simulink model "motor_new"  (R2018b)
settings: Solver=FixedStepAuto  StartTime=0.0  StopTime=100  FixedStep=0.001  RelTol=1e-3
values from neighbouring files (symbols this model uses):
  wt = 20    [Para_new.m]
libraries: simulink x2
settings Model: Creator=chengqian  LastModifiedBy=chengqian
settings SolverCC: AlgebraicLoopSolver=LineSearch

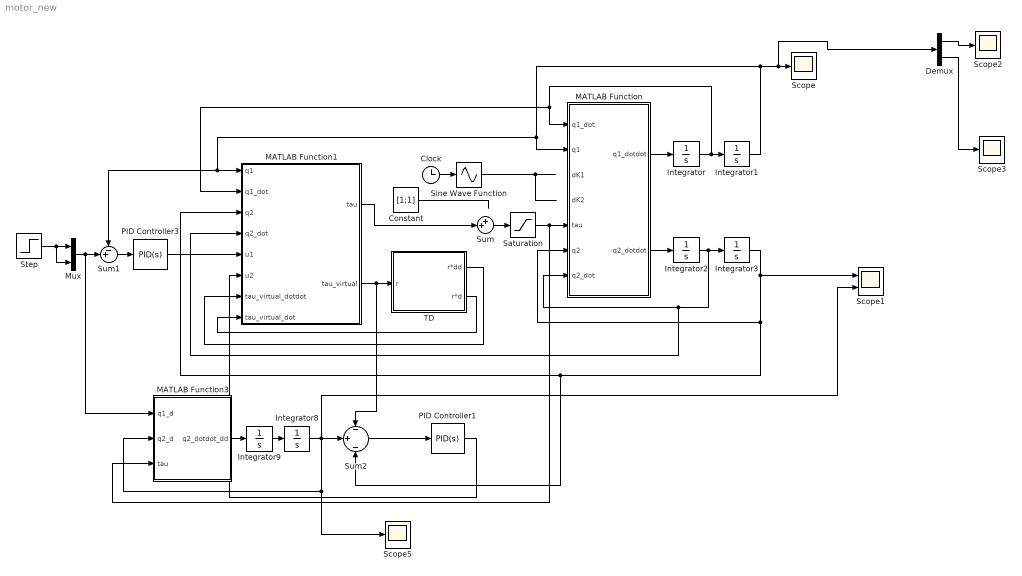
== system motor_new ==
  Clock : Clock
  Constant : Constant  Value=[1;1]
  Demux : Demux  Outputs=2
  Integrator{,1..3,8..9} (6 alike) : Integrator
  MATLAB Function : MATLAB Function  TreatAsAtomicUnit=on
  MATLAB Function1 : MATLAB Function  TreatAsAtomicUnit=on
  MATLAB Function3 : MATLAB Function  TreatAsAtomicUnit=on
  Mux : Mux  Inputs=2
  PID Controller1 : simulink/Continuous/PID Controller  Controller=PID  Form=Parallel  TimeDomain=Continuous-time  SampleTime=-1  IntegratorMethod=Forward Euler  FilterMethod=Forward Euler  ControllerParametersSource=internal  P=[0;0]  I=[0;0]  D=[0;0]  UseFilter=on  N=1000  TunerSelectOption=Transfer Function Based (PID Tuner App)  InitialConditionSource=internal  InitialConditionForIntegrator=0  InitialConditionForFilter=0  DifferentiatorICPrevScaledInput=0  ExternalReset=none  TrackingMode=off  Kt=1  LimitOutput=off  UpperSaturationLimit=inf  LowerSaturationLimit=-inf  LinearizeAsGain=on  AntiWindupMode=none  Kb=1  POutMin=[]  POutMax=[]  IOutMin=[]  IOutMax=[]  DOutMin=[]  DOutMax=[]  NOutMin=[]  NOutMax=[]  SumOutMin=[]  SumOutMax=[]  SaturationOutMin=[]  SaturationOutMax=[]  PParamMin=[]  PParamMax=[]  IParamMin=[]  IParamMax=[]  DParamMin=[]  DParamMax=[]  NParamMin=[]  NParamMax=[]  KbParamMin=[]  KbParamMax=[]  KtParamMin=[]  KtParamMax=[]  KbOutMin=[]  KbOutMax=[]  KtOutMin=[]  KtOutMax=[]  IntegratorOutMin=[]  IntegratorOutMax=[]  FilterOutMin=[]  FilterOutMax=[]  SumI1OutMin=[]  SumI1OutMax=[]  SumI2OutMin=[]  SumI2OutMax=[]  SumI3OutMin=[]  SumI3OutMax=[]  SumI4OutMin=[]  SumI4OutMax=[]  SumDOutMin=[]  SumDOutMax=[]  DifferentiatorOutMin=[]  DifferentiatorOutMax=[]  FilterDiffOutCoefMin=[]  FilterDiffOutCoefMax=[]  ReciprocalOutMin=[]  ReciprocalOutMax=[]  SumDenOutMin=[]  SumDenOutMax=[]  SumNumOutMin=[]  SumNumOutMax=[]  DivideOutMin=[]  DivideOutMax=[]  IntegratorContinuousStateAttributes=''  IntegratorStateMustResolveToSignalObject=off  IntegratorRTWStateStorageClass=Auto  FilterContinuousStateAttributes=''  FilterStateMustResolveToSignalObject=off  FilterRTWStateStorageClass=Auto  ParallelPVariant=InternalParameters  IdealPVariant=Disabled  IVariant=InternalParameters  DVariant=InternalParameters  IntegratorVariant=Continuous  SatVariant=Disabled  AWVariant=Passthrough  PCopyVariant=Disabled  TRVariant=Disabled  FdbkBlocksVariant=Forward  IdealPFdbkVariant=Disabled  SatFdbkVariant=Disabled  DerivativeFilterVariant=ContFilter  NVariant=InternalParameters  NCopyVariant=Disabled  FilterICVariant=InternalICsFilter  IntegratorICVariant=InternalICs  ExternalResetVariant=Disabled  TRSumVariant=Passthrough  SumFdbkVariant=Disabled  SumVariant=Sum_PID
  PID Controller3 : simulink/Continuous/PID Controller  Controller=PID  Form=Parallel  TimeDomain=Continuous-time  SampleTime=-1  IntegratorMethod=Forward Euler  FilterMethod=Forward Euler  ControllerParametersSource=internal  P=[2;2]  I=[0;0]  D=[0.1;0.05]  UseFilter=on  N=1000  TunerSelectOption=Transfer Function Based (PID Tuner App)  InitialConditionSource=internal  InitialConditionForIntegrator=0  InitialConditionForFilter=0  DifferentiatorICPrevScaledInput=0  ExternalReset=none  TrackingMode=off  Kt=1  LimitOutput=off  UpperSaturationLimit=inf  LowerSaturationLimit=-inf  LinearizeAsGain=on  AntiWindupMode=none  Kb=1  POutMin=[]  POutMax=[]  IOutMin=[]  IOutMax=[]  DOutMin=[]  DOutMax=[]  NOutMin=[]  NOutMax=[]  SumOutMin=[]  SumOutMax=[]  SaturationOutMin=[]  SaturationOutMax=[]  PParamMin=[]  PParamMax=[]  IParamMin=[]  IParamMax=[]  DParamMin=[]  DParamMax=[]  NParamMin=[]  NParamMax=[]  KbParamMin=[]  KbParamMax=[]  KtParamMin=[]  KtParamMax=[]  KbOutMin=[]  KbOutMax=[]  KtOutMin=[]  KtOutMax=[]  IntegratorOutMin=[]  IntegratorOutMax=[]  FilterOutMin=[]  FilterOutMax=[]  SumI1OutMin=[]  SumI1OutMax=[]  SumI2OutMin=[]  SumI2OutMax=[]  SumI3OutMin=[]  SumI3OutMax=[]  SumI4OutMin=[]  SumI4OutMax=[]  SumDOutMin=[]  SumDOutMax=[]  DifferentiatorOutMin=[]  DifferentiatorOutMax=[]  FilterDiffOutCoefMin=[]  FilterDiffOutCoefMax=[]  ReciprocalOutMin=[]  ReciprocalOutMax=[]  SumDenOutMin=[]  SumDenOutMax=[]  SumNumOutMin=[]  SumNumOutMax=[]  DivideOutMin=[]  DivideOutMax=[]  IntegratorContinuousStateAttributes=''  IntegratorStateMustResolveToSignalObject=off  IntegratorRTWStateStorageClass=Auto  FilterContinuousStateAttributes=''  FilterStateMustResolveToSignalObject=off  FilterRTWStateStorageClass=Auto  ParallelPVariant=InternalParameters  IdealPVariant=Disabled  IVariant=InternalParameters  DVariant=InternalParameters  IntegratorVariant=Continuous  SatVariant=Disabled  AWVariant=Passthrough  PCopyVariant=Disabled  TRVariant=Disabled  FdbkBlocksVariant=Forward  IdealPFdbkVariant=Disabled  SatFdbkVariant=Disabled  DerivativeFilterVariant=ContFilter  NVariant=InternalParameters  NCopyVariant=Disabled  FilterICVariant=InternalICsFilter  IntegratorICVariant=InternalICs  ExternalResetVariant=Disabled  TRSumVariant=Passthrough  SumFdbkVariant=Disabled  SumVariant=Sum_PID
  Saturation : Saturate  UpperLimit=[1000;1000]  LowerLimit=-[500;500]
  Scope{,2..3,5} (4 alike) : Scope
  Scope1 : Scope  NumInputPorts=2
  Sine Wave Function : Sin  TimeSource=Use external signal  Amplitude=0.4  Frequency=20  SampleTime=0
  Step : Step  Time=0  After=0.1  SampleTime=0
  Sum : Sum  Inputs=++|
  Sum1 : Sum  Inputs=-+|
  Sum2 : Sum  Inputs=-|+|-
  TD : Subsystem
  wires:
  MATLAB Function1/2(tau_virtual) -> Sum2/1, TD/1(r)
  MATLAB Function/1(q1_dotdot) -> Integrator/1
  Integrator/1 -> MATLAB Function/1(q1_dot), MATLAB Function1/2(q1_dot), Integrator1/1
  Integrator1/1 -> Demux/1, Scope/1, Sum1/1, MATLAB Function1/1(q1), MATLAB Function/2(q1)
  Integrator2/1 -> MATLAB Function1/4(q2_dot), MATLAB Function/7(q2_dot), Integrator3/1
  MATLAB Function/2(q2_dotdot) -> Integrator2/1
  Integrator3/1 -> MATLAB Function/6(q2), Sum2/3, MATLAB Function1/3(q2), Scope1/1
  MATLAB Function1/1(tau) -> Sum/2
  Clock/1 -> Sine Wave Function/1
  TD/2(r*d) -> MATLAB Function1/8(tau_virtual_dot)
  TD/1(r*dd) -> MATLAB Function1/7(tau_virtual_dotdot)
  Step/1 -> Mux/2, Mux/1
  Integrator8/1 -> Sum2/2, Scope1/2, Scope5/1, MATLAB Function3/2(q2_d)
  MATLAB Function3/1(q2_dotdot_dd) -> Integrator9/1
  Integrator9/1 -> Integrator8/1
  Sum1/1 -> PID Controller3/1
  Mux/1 -> Sum1/2, MATLAB Function3/1(q1_d)
  PID Controller3/1 -> MATLAB Function1/5(u1)
  Sum2/1 -> PID Controller1/1
  PID Controller1/1 -> MATLAB Function1/6(u2)
  Constant/1 -> ?
  Sine Wave Function/1 -> ?
  Sum/1 -> Saturation/1
  Saturation/1 -> MATLAB Function3/3(tau), MATLAB Function/5(tau)
  Demux/1 -> Scope2/1
  Demux/2 -> Scope3/1

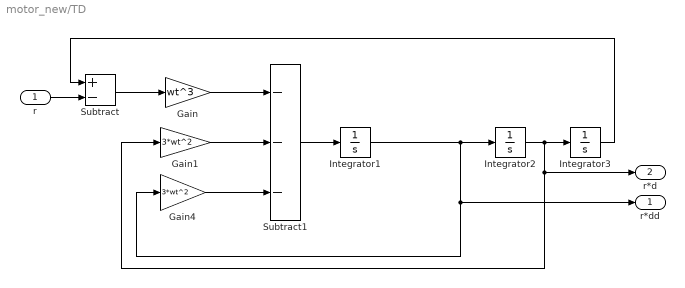
== system motor_new/TD ==
  r : Inport
  Gain : Gain  Gain=wt^3
  Gain1 : Gain  Gain=3*wt^2
  Gain4 : Gain  Gain=3*wt^2
  Integrator1 : Integrator
  Integrator2 : Integrator
  Integrator3 : Integrator
  Subtract : Sum  Inputs=+-
  Subtract1 : Sum  Inputs=---
  r*dd : Outport
  r*d : Outport  Port=2
  wires:
  Integrator2/1 -> Integrator3/1, Gain1/1, r*d/1
  Gain1/1 -> Subtract1/2
  Subtract/1 -> Gain/1
  Gain/1 -> Subtract1/1
  Integrator3/1 -> Subtract/1
  Gain4/1 -> Subtract1/3
  Subtract1/1 -> Integrator1/1
  Integrator1/1 -> Gain4/1, r*dd/1, Integrator2/1
  r/1 -> Subtract/2

== matlab function motor_new/MATLAB Function1 ==
  data: q1 input; tau output size=2; q1_dot input; q2 input; q2_dot input; u1 input; u2 input; tau_virtual_dotdot input; tau_virtual_dot input; tau_virtual output size=2
function [tau,tau_virtual] = fcn(q1,q1_dot,q2,q2_dot,u1,u2,tau_virtual_dotdot,tau_virtual_dot)

J11 = 3.17*10^(-4);
J22 = 0.97*10^(-4);
I1 = 0.96;
I2 = 0.71;
l1 = 0.6;
lc1 = 0.3;
lc2 = 0.5;
m1 = 19.31;
m2 = 13.73;
K1_ = 1.06*10^3;
K2_ = 0.75*10^3;
g = 9.8;

S11 = 1;
S12 = 1;
S21 = 2;
S22 = 2;
w1 =1;
beta1 = 2; beta2 = 2;
alpha1 = 10; alpha2 = 10;
Kp1 = 100; Kd1 =20;

dK1=0;dK2=0;

q11 = q1(1);
q12 = q1(2);
q11_dot = q1_dot(1);
q12_dot = q1_dot(2);

q21 = q2(1);
q22 =q2(2);
q21_dot = q2_dot(1);
q22_dot = q2_dot(2);

M11 = m2*(l1^2 + lc2^2 + 2*l1*lc2*cos(q12)) + m1*lc1^2 + I1 + I2;
M12 = m2*(lc2^2 + l1*lc2*cos(q12)) + I2;
M21 = M12;
M22 = m2*lc2^2 + I2;

M = [M11,M12;M21,M22];

C11 = -m1*l1*lc2*sin(q12)*q12_dot;
C12 = -m2*l1*lc2*sin(q12)*(q11_dot + q12_dot);
C21 = m2*l1*lc2*sin(q12)*q11_dot;
C22 = 0;

C = [C11,C12;C21,C22];

G1 = (m1*lc1 + m2*l1)*g*sin(q11) + m2*lc2*g*sin(q11 + q12);
G2 = m2*lc2*g*sin(q11+q12);

G = [G1;G2];

J = diag([J11,J22]);
S1 = diag([S11,S12]);
S2 = diag([S21,S22]);
K_ = diag([K1_,K2_]);
K = diag([K1_,K2_])*(eye(2) + diag([dK1,dK2]));

M11_dot = -2*m2*l1*lc2*sin(q12)*q12_dot;
M12_dot = -m2*l1*lc2*sin(q12)*q12_dot;
M21_dot = -m2*l1*lc2*sin(q11)*q12_dot;
M22_dot = 0;

M_dot = [M11_dot,M12_dot;M21_dot,M22_dot];

PHI1 = 0.5*M_dot*(q1_dot + S1*q1) - C*q1_dot - G -K_*q1 + M*S1*q1_dot;
rol1_bound = norm(PHI1);
rol1 = 0;

% if rol1>rol1_bound
%     rol1 = rol1_bound;
% else
%     rol1 = 0;
% end

tau_virtual =K_'* u1;% + K_'*(Kp1*q1_r - Kp1*q1 - Kd1*q1_dot));(K_'*(-alpha1*(q1_dot + S1*q1)*rol1^2 - beta1*(q1_dot + S1*q1)) + 
x3 = q2 - tau_virtual;
x4 = q2_dot - tau_virtual_dot;
PHI2 = -J*tau_virtual_dotdot - K_*(x3) + K_*q1 - K_*tau_virtual + J*S2*x4;
rol2_bound = norm(PHI2);
rol2 = rol2_bound;

% if rol2>rol2_bound
%     rol2 = rol2_bound;
% else
%     rol2 = 0;
% end

tau =(-alpha2*(x4+S2*x3)*rol2^2 - beta2*(x4+S2*x3)) + u2;% + (-Kp1*x3 - Kd1*x4); + 
%q2_dotdot_dd = J'*(tau + K*(q1_d - q2_d));

== matlab function motor_new/MATLAB Function ==
  data: q1_dot input; q1 input; dK1 input; dK2 input; q1_dotdot output size=2; tau input; q2 input; q2_dot input; q2_dotdot output size=2
function [q1_dotdot,q2_dotdot] = fcn(q1_dot,q1,dK1,dK2,tau,q2,q2_dot)
J11 = 3.17*10^(-4);
J22 = 0.97*10^(-4);
I1 = 0.96;
I2 = 0.71;
l1 = 0.6;
lc1 = 0.3;
lc2 = 0.5;
m1 = 19.31;
m2 = 13.73;
K1_ = 1.06*10^3;
K2_ = 0.75*10^3;
g = 9.8;

S11 = 1;
S12 = 1;
S21 = 2;
S22 = 2;
w1 =1;
beta1 = 2; beta2 = 2;
alpha1 = 10; alpha2 = 10;
Kp1 = 100; Kd1 =20;


q11 = q1(1);
q12 = q1(2);
q11_dot = q1_dot(1);
q12_dot = q1_dot(2);

q21 = q2(1);
q22 =q2(2);
q21_dot = q2_dot(1);
q22_dot = q2_dot(2);

M11 = m2*(l1^2 + lc2^2 + 2*l1*lc2*cos(q12)) + m1*lc1^2 + I1 + I2;
M12 = m2*(lc2^2 + l1*lc2*cos(q12)) + I2;
M21 = M12;
M22 = m2*lc2^2 + I2;

M = [M11,M12;M21,M22];

C11 = -m1*l1*lc2*sin(q12)*q12_dot;
C12 = -m2*l1*lc2*sin(q12)*(q11_dot + q12_dot);
C21 = m2*l1*lc2*sin(q12)*q11_dot;
C22 = 0;

C = [C11,C12;C21,C22];

G1 = (m1*lc1 + m2*l1)*g*sin(q11) + m2*lc2*g*sin(q11 + q12);
G2 = m2*lc2*g*sin(q11+q12);

G = [G1;G2];

J = diag([J11,J22]);
S1 = diag([S11,S12]);
S2 = diag([S21,S22]);
K = diag([K1_,K2_])*(eye(2) + diag([dK1,dK2]));

q1_dotdot = -M'*(C*q1_dot + G + K*(q1-q2));
q2_dotdot = J'*(tau + K*(q1-q2));

== matlab function motor_new/MATLAB Function3 ==
  data: q1_d input; q2_dotdot_dd output; q2_d input; tau input
function q2_dotdot_dd = fcn(q1_d,q2_d,tau)
J11 = 3.17*10^(-4);
J22 = 0.97*10^(-4);
J = diag([J11,J22]);

K1_ = 1.06*10^3;
K2_ = 0.75*10^3;

K_ = diag([K1_,K2_]);


q2_dotdot_dd = J'*(tau + K_*(q1_d - q2_d));
